simulink library "lib_Conduction_HeatX1DVarPropsAndGenBCs"  (R2015a)
settings: Solver=ode45  StartTime=0.0  StopTime=10.0  RelTol=1e-3
undefined symbols (not defined in the file): dt, T0, x
settings Model: Creator=jlkratz  LastModifiedBy=jlkratz

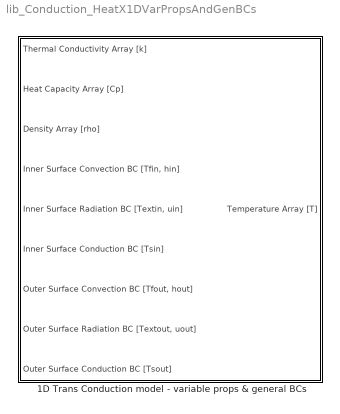
== system lib_Conduction_HeatX1DVarPropsAndGenBCs ==
  1D Trans Conduction model - variable props & general BCs : Subsystem  mask(TSAT: 1-D Trans Conduction Model - Variable Props + Generic BCs Block){x_M=x, T0_M=T0, dt_M=dt, a_M=on, convin_M=on, radin_M=on, condin_M=on, convout_M=on, radout_M=on, condout_M=on, BN_M=double(gcb)}
      mask prompts: x_M "x_M - Discretized spatial domain (node locations) (nx1 array)"; T0_M "T0_M - Initial temperature array (nx1 array)"; dt_M "dt_M - Time step"; a_M "a_M - Shape (unchecked - planar, checked - cylindrical)"; convin_M "convin_M - Convection"; radin_M "radin_M - Radiation"; condin_M "condin_M - Conduction"; convout_M "convout_M - Convection"; radout_M "radout_M - Radiation"; condout_M "condout_M- Conduction"; BN_M "BN_M - Block name"
      mask help:
      | This function models the transient conduction of a 1-D structure which can either be of a planar or cylindrical geometry. This block solves the general 1-D heat equation using a finite difference method. It is able to handle variable thermal properties including density, heat capacity, and thermal conductivity. Abrupt transitions in material are also considered. It has the capability to address dynamic convection, conduction, and radiation boundary conditions. In addition, the discretized domain can be non-uniform but with the restriction that the boundary nodes should be half the thickness of their neighboring interior node (see the help menu).
      |
      | This block is able to accept inputs and parameters in a variety of units but it is important that the units be consistent. More details about this function, it's parameters, inputs, and outputs are provided in the help menu of this block.
      mask init:
      | % Setup Inports ----------------------------------------------------------%
      | 
      | % Inport Numbers
      | n = 4; %first BC inport number
      | 
      | % Inner Suface Convection Boundary Condition
      | if convin_M == 1
      |     if strcmp(get_param([BN_M '/Inner Surface Convection BC [Tfin, hin]'],'BlockType'),'Constant')
      |         MSK_ReplaceBlock_TSAT([BN_M '/Inner Surface Convection BC [Tfin, hin]'],'built-in/Inport');
      |     end
      |     set_param([BN_M '/Inner Surface Convection BC [Tfin, hin]'],'Port',num2str(n));
      |     n = n + 1;
      | elseif convin_M == 0
      |     if strcmp(get_param([BN_M '/Inner Surface Convection BC [Tfin, hin]'],'BlockType'),'Inport')
      |         MSK_ReplaceBlock_TSAT([BN_M '/Inner Surface Convection BC [Tfin, hin]'],'built-in/Constant');
      |         set_param([BN_M '/Inner Surface Convection BC [Tfin, hin]'],'Value','[0, 0]');
      |     end
      | end
      | 
      | % Inner Suface Radiation Boundary Condition
      | if radin_M == 1
      |     if strcmp(get_param([BN_M '/Inner Surface Radiation BC [Textin, uin]'],'BlockType'),'Constant')
      |         MSK_ReplaceBlock_TSAT([BN_M '/Inner Surface Radiation BC [Textin, uin]'],'built-in/Inport');
      |     end
      |     set_param([BN_M '/Inner Surface Radiation BC [Textin, uin]'],'Port',num2str(n));
      |     n = n + 1;
      | elseif radin_M == 0
      |     if strcmp(get_param([BN_M '/Inner Surface Radiation BC [Textin, uin]'],'BlockType'),'Inport')
      |         MSK_ReplaceBlock_TSAT([BN_M '/Inner Surface Radiation BC [Textin, uin]'],'built-in/Constant');
      |         set_param([BN_M '/Inner Surface Radiation BC [Textin, uin]'],'Value','[0, 0]');
      |     end
      | end
      | 
      | % Inner Suface Conduction Boundary Condition
      | if condin_M == 1
      |     if strcmp(get_param([BN_M '/Inner Surface Conduction BC [Tsin]'],'BlockType'),'Constant')
      |         MSK_ReplaceBlock_TSAT([BN_M '/Inner Surface Conduction BC [Tsin]'],'built-in/Inport');
      |     end
      |     set_param([BN_M '/Inner Surface Conduction BC [Tsin]'],'Port',num2str(n));
      |     n = n + 1;
      | elseif condin_M == 0
      |     if strcmp(get_param([BN_M '/Inner Surface Conduction BC [Tsin]'],'BlockType'),'Inport')
      |         MSK_ReplaceBlock_TSAT([BN_M '/Inner Surface Conduction BC [Tsin]'],'built-in/Constant');
      |         set_param([BN_M '/Inner Surface Conduction BC [Tsin]'],'Value','0');
      |     end
      | end
      | 
      | % Outer Suface Convection Boundary Condition
      | if convout_M == 1
      |     if strcmp(get_param([BN_M '/Outer Surface Convection BC [Tfout, hout]'],'BlockType'),'Constant')
      |         MSK_ReplaceBlock_TSAT([BN_M '/Outer Surface Convection BC [Tfout, hout]'],'built-in/Inport');
      |     end
      |     set_param([BN_M '/Outer Surface Convection BC [Tfout, hout]'],'Port',num2str(n));
      |     n = n + 1;
      | elseif convout_M == 0
      |     if strcmp(get_param([BN_M '/Outer Surface Convection BC [Tfout, hout]'],'BlockType'),'Inport')
      |         MSK_ReplaceBlock_TSAT([BN_M '/Outer Surface Convection BC [Tfout, hout]'],'built-in/Constant');
      |         set_param([BN_M '/Outer Surface Convection BC [Tfout, hout]'],'Value','[0, 0]');
      |     end
      | end
      | 
      | % Outer Suface Radiation Boundary Condition
      | if radout_M == 1
      |     if strcmp(get_param([BN_M '/Outer Surface Radiation BC [Textout, uout]'],'BlockType'),'Constant')
      |         MSK_ReplaceBlock_TSAT([BN_M '/Outer Surface Radiation BC [Textout, uout]'],'built-in/Inport');
      |     end
      |     set_param([BN_M '/Outer Surface Radiation BC [Textout, uout]'],'Port',num2str(n));
      |     n = n + 1;
      | elseif radout_M == 0
      |     if strcmp(get_param([BN_M '/Outer Surface Radiation BC [Textout, uout]'],'BlockType'),'Inport')
      |         MSK_ReplaceBlock_TSAT([BN_M '/Outer Surface Radiation BC [Textout, uout]'],'built-in/Constant');
      |         set_param([BN_M '/Outer Surface Radiation BC [Textout, uout]'],'Value','[0, 0]');
      |     end
      | end
      | 
      | % Outer Suface Conduction Boundary Condition
      | if condout_M == 1
      |     if strcmp(get_param([BN_M '/Outer Surface Conduction BC [Tsout]'],'BlockType'),'Constant')
      |         MSK_ReplaceBlock_TSAT([BN_M '/Outer Surface Conduction BC [Tsout]'],'built-in/Inport');
      |     end
      |     set_param([BN_M '/Outer Surface Conduction BC [Tsout]'],'Port',num2str(n));
      |     n = n + 1;
      | elseif condout_M == 0
      |     if strcmp(get_param([BN_M '/Outer Surface Conduction BC [Tsout]'],'BlockType'),'Inport')
      |         MSK_ReplaceBlock_TSAT([BN_M '/Outer Surface Conduction BC [Tsout]'],'built-in/Constant');
      |         set_param([BN_M '/Outer Surface Conduction BC [Tsout]'],'Value','0');
      |     end
      | end
      mask Help: web(which('Conduction_TSAT_1DTCondVarPropGenBC.html'),'-helpbrowser')
      mask DialogControl Container3 Prompt: General Parameters
      mask DialogControl Container4 Prompt: Active Inner Boundary Conditions
      mask DialogControl Container7 Prompt: Active Outer Boundary Conditions

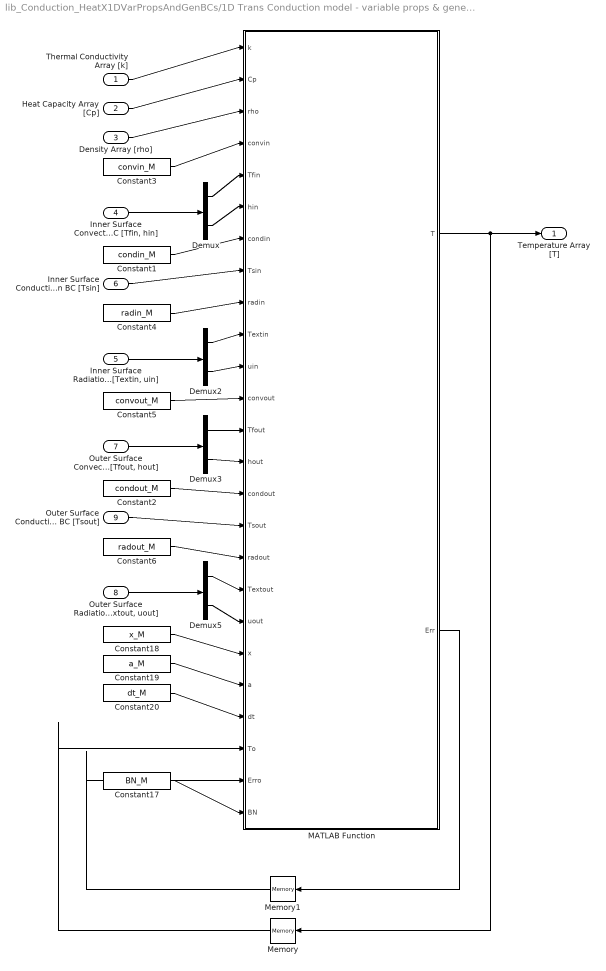
== system lib_Conduction_HeatX1DVarPropsAndGenBCs/1D Trans Conduction model - variable props & general BCs ==
  Thermal Conductivity Array [k] : Inport
  Heat Capacity Array [Cp] : Inport  Port=2
  Density Array [rho] : Inport  Port=3
  "Inner Surface Convection BC [Tfin, hin]" : Inport  Port=4
  "Inner Surface Radiation BC [Textin, uin]" : Inport  Port=5
  Inner Surface Conduction BC [Tsin] : Inport  Port=6
  "Outer Surface Convection BC [Tfout, hout]" : Inport  Port=7
  "Outer Surface Radiation BC [Textout, uout]" : Inport  Port=8
  Outer Surface Conduction BC [Tsout] : Inport  Port=9
  Constant1 : Constant  Value=condin_M
  Constant17 : Constant  Value=BN_M
  Constant18 : Constant  Value=x_M
  Constant19 : Constant  Value=a_M
  Constant2 : Constant  Value=condout_M
  Constant20 : Constant  Value=dt_M
  Constant3 : Constant  Value=convin_M
  Constant4 : Constant  Value=radin_M
  Constant5 : Constant  Value=convout_M
  Constant6 : Constant  Value=radout_M
  Demux{,2..3,5} (4 alike) : Demux  Outputs=[1 1]
  MATLAB Function : MATLAB Function  TreatAsAtomicUnit=on
  Memory : Memory  X0=T0_M
  Memory1 : Memory  X0=zeros(1,37)
  Temperature Array [T] : Outport
  wires:
  "Outer Surface Radiation BC [Textout, uout]"/1 -> Demux5/1
  Demux5/2 -> MATLAB Function/19(uout)
  Demux5/1 -> MATLAB Function/18(Textout)
  Outer Surface Conduction BC [Tsout]/1 -> MATLAB Function/16(Tsout)
  Demux3/2 -> MATLAB Function/14(hout)
  Demux3/1 -> MATLAB Function/13(Tfout)
  "Outer Surface Convection BC [Tfout, hout]"/1 -> Demux3/1
  Demux2/2 -> MATLAB Function/11(uin)
  Demux2/1 -> MATLAB Function/10(Textin)
  "Inner Surface Radiation BC [Textin, uin]"/1 -> Demux2/1
  Inner Surface Conduction BC [Tsin]/1 -> MATLAB Function/8(Tsin)
  Demux/2 -> MATLAB Function/6(hin)
  Demux/1 -> MATLAB Function/5(Tfin)
  "Inner Surface Convection BC [Tfin, hin]"/1 -> Demux/1
  Constant6/1 -> MATLAB Function/17(radout)
  Constant5/1 -> MATLAB Function/12(convout)
  Constant4/1 -> MATLAB Function/9(radin)
  Constant3/1 -> MATLAB Function/4(convin)
  Constant2/1 -> MATLAB Function/15(condout)
  Constant1/1 -> MATLAB Function/7(condin)
  MATLAB Function/2(Err) -> Memory1/1
  Memory/1 -> MATLAB Function/23(To)
  MATLAB Function/1(T) -> Temperature Array [T]/1, Memory/1
  Constant20/1 -> MATLAB Function/22(dt)
  Constant19/1 -> MATLAB Function/21(a)
  Constant18/1 -> MATLAB Function/20(x)
  Density Array [rho]/1 -> MATLAB Function/3(rho)
  Heat Capacity Array [Cp]/1 -> MATLAB Function/2(Cp)
  Thermal Conductivity Array [k]/1 -> MATLAB Function/1(k)
  Memory1/1 -> MATLAB Function/24(Erro)
  Constant17/1 -> MATLAB Function/25(BN)

== matlab function lib_Conduction_HeatX1DVarPropsAndGenBCs/1D Trans Conduction model - variable props & general BCs/MATLAB Function ==
  data: k input; T output; Cp input; rho input; convin input; Tfin input; hin input; condin input; Tsin input; radin input; Textin input; uin input; convout input; Tfout input; hout input; condout input; Tsout input; radout input; Textout input; uout input; x input; a input; dt input; To input; Erro input; Err output; BN input
function [T,Err] = HeatX1D(k,Cp,rho,convin,Tfin,hin,condin,Tsin,...
    radin,Textin,uin,convout,Tfout,hout,condout,Tsout,radout,Textout,uout,...
    x,a,dt,To,Erro,BN)
%#codegen

% Written by: Jonathan Kratz, NASA GRC
% Date: August 1, 2016
%
% Description: This MATLAB function block solves a 1-D heat transfer
% problem with the potential for various boundary conditions including
% convection, conduction, and radiation. The function is capable of
% accepting time-varying thermal properties including the conductivity,
% specific heat, and density of the solid structure. Heat transfer
% coefficients can also be time-varying. The function is equiped to handle
% planor and cylindrical geometries. A generic non-uniform spatial
% discretization may be used but a constant time-step is encouraged for
% accuracy in time. The block applies a 1-D Finite Difference Method (FDM)
% to solve the equation:
%                  _                     _
%   dT     1      |  /dk   ak\ dT     d2T |
%   -- = ------ * | | -- + -- |-- + k --- |
%   dt   rho*Cp   |_ \dx    x/ dx     dx2_|
%
% This is done through the Crank-Nicolson Method in conjunction with 
% Thomas's Algorithm. The boundary conditions use linear heat transfer 
% coefficients and it is suggested that these coefficients be evaluated 
% using thermal properties of the previous time-step (i.e. temperature of 
% the structure and thermodynamic properties of the surrounding gases).
% Depending on the problem they may be assumed constant.
%
% Inputs:
% Thermal Properties:
%   k - thermal conductivity of the structure [1 x number of nodes]
%   Cp - heat capacity of the structure [1 x number of nodes]
%   rho - density of the structure [1 x number of nodes]
% Boundary Conditions:
%   Tfin - temperature of fluid on the inside surface
%   hin - convective heat transfer coefficient on the inside surface
%   Tsin - temperature of a contacting structure on the inside surface
%   Textin - temperature of a distant external radiating source/sink 
%       exposed to the inner surface
%   uin - linear radiative heat transfer coefficient between the inner
%       surface and external radiating source/sink it is exposed to
%   Tfout - temperature of fluid on the outer surface
%   hout - convective heat transfer coefficient on the outer surface
%   Tsout - temperature of a contacting structure on the outer surface
%   Textout - temperature of a distant external radiating source/sink 
%       exposed to the outer surface
%   uin - linear radiative heat transfer coefficient between the outer
%       surface and external radiating source/sink it is exposed to
% Geometry/Discretization:
%   x - discretized spatial coordinates
%   a - shape variable (0 - planar, 1 - cylindrical)
% Solver:
%   dt - time-step of the solver
%   To - initial condition for the solver/initial temperature of the
%       structure [1 x number of nodes]
% Error/Warning Detection
%   Erro - array with error states. Tracks errors/warnings that have been
%       detected.
%   BN - block name. Used in warning messages.
%  
% Discretization guidelines: The first and last nodes should be on the 
% surface. It is important that that the first node should be half the size 
% as the second node and the last node should be half the size of the 
% second to last node. This is due to the assumptions made in the 
% formulization of the boundary condition equations. Also, for planar 
% geometries the first value of the discretization array x (which 
% corresponds to the first node) can be any real numeric value (it does not
% have to be zero, equations use node size so relative position is what 
% matters). In the case of a cylindrical geometry the first value in the x 
% array should be the inner radius of the structure. It should go without 
% saying that the spatial discretization array x is required to be 
% montonically increasing.

% number of elements
n = length(x); %number of nodes

% initialize error/warning array
Err = Erro;
ErrNum = 1; %Error index

% check sizes ------------------------------------------------------------%
if length(x) < 4 && Erro(ErrNum) == 0
    Err(ErrNum) = 1;
    fprintf('warning in %s: x must be an array of length > 3\n',char(BN));
end
ErrNum = ErrNum + 1;
if length(k) ~= length(x) && Erro(ErrNum) == 0
    Err(ErrNum) = 1;
    fprintf('warning in %s: length of k must equal length of x\n',char(BN));
end
ErrNum = ErrNum + 1;
if length(Cp) ~= length(x) && Erro(ErrNum) == 0
    Err(ErrNum) = 1;
    fprintf('warning in %s: length of k must equal length of x\n',char(BN));
end
ErrNum = ErrNum + 1;
if length(rho) ~= length(x) && Erro(ErrNum) == 0
    Err(ErrNum) = 1;
    fprintf('warning in %s: length of k must equal length of x\n',char(BN));
end
ErrNum = ErrNum + 1;
if length(x) ~= length(x) && Erro(ErrNum) == 0
    Err(ErrNum) = 1;
    fprintf('warning in %s: length of k must equal length of x\n',char(BN));
end
ErrNum = ErrNum + 1;
if length(Tfin) ~= 1 && Erro(ErrNum) == 0
    Err(ErrNum) = 1;
    fprintf('warning in %s: Tfin must be a scalar\n',char(BN));
end
ErrNum = ErrNum + 1;
if length(hin) ~= 1 && Erro(ErrNum) == 0
    Err(ErrNum) = 1;
    fprintf('warning in %s: hin must be a scalar\n',char(BN));
end
ErrNum = ErrNum + 1;
if length(Tsin) ~= 1 && Erro(ErrNum) == 0
    Err(ErrNum) = 1;
    fprintf('warning in %s: Tsin must be a scalar\n',char(BN));
end
ErrNum = ErrNum + 1;
if length(Textin) ~= 1 && Erro(ErrNum) == 0
    Err(ErrNum) = 1;
    fprintf('warning in %s: Textin must be a scalar\n',char(BN));
end
ErrNum = ErrNum + 1;
if length(uin) ~= 1 && Erro(ErrNum) == 0
    Err(ErrNum) = 1;
    fprintf('warning in %s: uin must be a scalar\n',char(BN));
end
ErrNum = ErrNum + 1;
if length(Tfout) ~= 1 && Erro(ErrNum) == 0
    Err(ErrNum) = 1;
    fprintf('warning in %s: Tfout must be a scalar\n',char(BN));
end
ErrNum = ErrNum + 1;
if length(hout) ~= 1 && Erro(ErrNum) == 0
    Err(ErrNum) = 1;
    fprintf('warning in %s: hout must be a scalar\n',char(BN));
end
ErrNum = ErrNum + 1;
if length(Tsout) ~= 1 && Erro(ErrNum) == 0
    Err(ErrNum) = 1;
    fprintf('warning in %s: Tsout must be a scalar\n',char(BN));
end
ErrNum = ErrNum + 1;
if length(Textout) ~= 1 && Erro(ErrNum) == 0
    Err(ErrNum) = 1;
    fprintf('warning in %s: Textout must be a scalar\n',char(BN));
end
ErrNum = ErrNum + 1;
if length(uout) ~= 1 && Erro(ErrNum) == 0
    Err(ErrNum) = 1;
    fprintf('warning in %s: uin must be a scalar\n',char(BN));
end
ErrNum = ErrNum + 1;
if ((length(a) ~= 1) || (a ~= 0 && a ~= 1)) && Erro(ErrNum) == 0
    Err(ErrNum) = 1;
    fprintf('warning in %s: a must be a scalar equal to 0 or 1\n',char(BN));
end
ErrNum = ErrNum + 1;
if (length(dt) ~= 1 || dt <= 0) && Erro(ErrNum) == 0
    Err(ErrNum) = 1;
    fprintf('warning in %s: dt must be a positive scalar\n',char(BN));
end
ErrNum = ErrNum + 1;

% check for physical impossibilities
if min(k) <= 0 && Erro(ErrNum) == 0
    Err(ErrNum) = 1;
    fprintf('warning in %s: elements of k cannot be zero or negative\n',char(BN));
end
ErrNum = ErrNum + 1;
if min(Cp) <= 0 && Erro(ErrNum) == 0
    Err(ErrNum) = 1;
    fprintf('warning in %s: elements of Cp cannot be zero or negative\n',char(BN));
end
ErrNum = ErrNum + 1;
if min(rho) <= 0 && Erro(ErrNum) == 0
    Err(ErrNum) = 1;
    fprintf('warning in %s: elements of rho cannot be zero or negative\n',char(BN));
end
ErrNum = ErrNum + 1;
if min(To) < 0 && Erro(ErrNum) == 0
    Err(ErrNum) = 1;
    fprintf('warning in %s: elements of T0 are negative. On an absolute scale this is not possible.\n',char(BN));
end
ErrNum = ErrNum + 1;
if Tfin < 0 && Erro(ErrNum) == 0
    Err(ErrNum) = 1;
    fprintf('warning in %s: Tfin is negative. On an absolute scale this is not possible.\n',char(BN));
end
ErrNum = ErrNum + 1;
if Tfout < 0 && Erro(ErrNum) == 0
    Err(ErrNum) = 1;
    fprintf('warning in %s: Tfout is negative. On an absolute scale this is not possible.\n',char(BN));
end
ErrNum = ErrNum + 1;
if Tsin < 0 && Erro(ErrNum) == 0
    Err(ErrNum) = 1;
    fprintf('warning in %s: Tsin is negative. On an absolute scale this is not possible.\n',char(BN));
end
ErrNum = ErrNum + 1;
if Tsout < 0 && Erro(ErrNum) == 0
    Err(ErrNum) = 1;
    fprintf('warning in %s: Tsout is negative. On an absolute scale this is not possible.\n',char(BN));
end
ErrNum = ErrNum + 1;
if Textin < 0 && Erro(ErrNum) == 0
    Err(ErrNum) = 1;
    fprintf('warning in %s: Textin is negative. On an absolute scale this is not possible.\n',char(BN));
end
ErrNum = ErrNum + 1;
if Textout < 0 && Erro(ErrNum) == 0
    Err(ErrNum) = 1;
    fprintf('warning in %s: Textout is negative. On an absolute scale this is not possible.\n',char(BN));
end
ErrNum = ErrNum + 1;
if hin < 0 && Erro(ErrNum) == 0
    Err(ErrNum) = 1;
    fprintf('warning in %s: hin must be positive.\n',char(BN));
end
ErrNum = ErrNum + 1;
if hout < 0 && Erro(ErrNum) == 0
    Err(ErrNum) = 1;
    fprintf('warning in %s: hout must be positive.\n',char(BN));
end
ErrNum = ErrNum + 1;
if uin < 0 && Erro(ErrNum) == 0
    Err(ErrNum) = 1;
    fprintf('warning in %s: uin must be positive.\n',char(BN));
end
ErrNum = ErrNum + 1;
if uout < 0 && Erro(ErrNum) == 0
    Err(ErrNum) = 1;
    fprintf('warning in %s: uout must be positive.\n',char(BN));
end
ErrNum = ErrNum + 1;

% check for defiance of block constraints
diffx = diff(x);
if min(diffx) <= 0 && Erro(ErrNum) == 0
    Err(ErrNum) = 1;
    fprintf('warning in %s: x must be monotonically increasing\n',char(BN));
end
ErrNum = ErrNum + 1;
if (x(2)-x(1))-(x(3)-x(2)) >= 10^-5 && Erro(ErrNum) == 0
    x(1)
    x(2)
    x(3)
    Err(ErrNum) = 1;
    fprintf('warning in %s: the first node may not be half the thickness of the\nneighboring interior node as is required for planar geometries in the\nequation formulation of this block. To assure the first node is\nof the appropriate size assure (x(2)-x(1))-(x(3)-x(2)) = 0.\n',char(BN));
end
ErrNum = ErrNum + 1;
if (x(n)-x(n-1))-(x(n-1)-x(n-2)) >= 10^-5 && Erro(ErrNum) == 0
    Err(ErrNum) = 1;
    fprintf('warning in %s: the last node may not be half the thickness of the\nneighboring interior node as is required for planar geometries in the\nequation formulation of this block. To assure the last node is\nof the appropriate size assure (x(n)-x(n-1))-(x(n-1)-x(n-2)) = 0\nwhere n is the total number of nodes.\n',char(BN));
end
ErrNum = ErrNum + 1;
if a == 1 && x(1) < 10^-6 %protect against dividing by zero
    if Erro(ErrNum) == 0
        fprintf('warning in %s: x(1) is close to zero, value changed to 10^-6 to prevent dividing by zero\n',char(BN));
    end
    Err(ErrNum) = 1;
    x(1) = 10^-6;
end
ErrNum = ErrNum + 1;

% verify at least one BC type is active for each surface
if condin == 0 && convin == 0 && radin == 0 && Erro(ErrNum) == 0
    fprintf('warning in %s: at least one boundary condition type (convection, radiation, conduction) must be active for the inner surface\n',char(BN));
    Err(ErrNum) = 1;
end
ErrNum = ErrNum + 1;
% verify at least one BC type is active for each surface
if condout == 0 && convout == 0 && radout == 0 && Erro(ErrNum) == 0
    fprintf('warning in %s: at least one boundary condition type (convection, radiation, conduction) must be active for the outer surface\n',char(BN));
    Err(ErrNum) = 1;
end

% make external convection at boundaries zero if there is no convection BC
if convin == 0
    hin = 0;
end
if convout == 0
    hout = 0;
end

% make external radiation at boundaries zero if there is no radiation BC
if radin == 0
    uin = 0;
end
if radout == 0
    uout = 0;
end

% form system of equations in tridiagonal arrays -------------------------%
%  _                                 _  _   _     _   _ 
% | D1   A1   0    .    .    .    0   || T1  |   | C1  |
% | B1   D2   A2   0              .   || T2  |   | C2  |
% | 0    B2   D3   A3   .         .   || T3  |   | C3  |
% | .    0    .    .    .    .    .   || .   | = | .   |
% | .         .    .    .    .    0   || .   |   | .   | 
% | .              .    Bn-2 Dn-1 An-1|| Tn-1|   | Cn-1|
% |_0    .    .    .    0    Bn-1 Dn _||_Tn _|   |_Cn _|
%
% Initialize system arrays B, D, A, and C
B = zeros(1,n); %initialize B array
D = zeros(1,n); %initialize D array
A = zeros(1,n); %initialize A array
C = zeros(1,n); %initialize C array
% node thickness
dx = zeros(1,n); %initialize dx array
for i = 1:n
    if i == 1
        dx(i) = (x(2)-x(1));
    elseif i == n
        dx(i) = (x(n)-x(n-1));
    else
        del1 = x(i) - x(i-1);
        dx(i) = 2*del1 - dx(i-1);
    end
end
% --- inner node (half size of interior node with point on surface)
Fo1 = 0; %Fourier number
Bi1 = 0; %Boit number
BiRad1 = 0; %analogous Boit number for radiation
Fos1 = 0; %Fourier number for conduction BC
dx1 = x(2) - x(1); %node size
% planar
if a == 0
    Fo1 = dt*k(1)/(rho(1)*Cp(1)*dx1^2); %Fourier number
    Bi1 = hin*dx1/k(1); %Boit number
    BiRad1 = uin*dx1/k(1); %analogous Boit number for radiation
    if condin == 0
        Fos1 = 0;
    else
        Fos1 = Fo1/(10^-4); %Fourier number for conduction BC
    end
end
% cylindrical
if a == 1
    Fo1 = dt*k(1)/(rho(1)*Cp(1)*((x(2)-dx1/2)^2-x(1)^2)*log(x(2)/x(1))); %Fourier number
    Bi1 = hin*x(1)*log(x(2)/x(1))/k(1); %Boit number
    BiRad1 = uin*x(1)*log(x(2)/x(1))/k(1); %analogous Boit number for radiation
    if condin == 0
        Fos1 = 0;
    else
        if (x(1)-dx1) <= 0
            dx1 = 0;
        end
        Fos1 = dt*k(1)/(rho(1)*Cp(1)*((x(2)-dx1/2)^2-x(1)^2)*log((x(1)/(x(1)-dx1))))/(10^-4); %Fourier number for conduction BC
    end
end
% form system arrays
B(1) = 0;
D(1) = 1 + Fo1 + Fo1*Bi1 + Fo1*BiRad1 + Fos1; %system array D
A(1) = -Fo1; %system array A
C(1) = (1 - Fo1 - Fo1*Bi1 - Fo1*BiRad1 - Fos1)*To(1) + Fo1*To(2) + 2*Fo1*Bi1*Tfin + 2*Fo1*BiRad1*Textin + 2*Fos1*Tsin; %system array C
% --- interior nodes
for i = 2:(n-1)
    % distance between nodes
    del1 = x(i) - x(i-1);
    del2 = x(i+1) - x(i);
    % simplification coefficients (for spatial discretization)
    C1 = 1 + (del1^3/del2^2 - del1)/(del2 + del1);
    C2 = 1 + (del1/del2)^3;
    C3 = (del1/del2)^3 - ((del1^3/del2^2) - del1)/(del2+del1);
    % calculated Fourier numbers
    Fo = 2*k(i)*dt/(rho(i)*Cp(i)*(del1^2 + del1^3/del2)); %Fourier number
    Fok = (dt/(rho(i)*Cp(i)*(del1+del2)))*((k(i+1)-k(i-1))/(del1+del2) + a*k(i)/x(i)); %Fourier number for conductivity variation and shape
    % adjust equations for change in materials
    %   when there is a change in materials the transition in materials
    %   properties, most notabely thermal conductivity, is abrupt. This
    %   discontinuty can cause accuracy and stability issues with the 
    %   derivative term dk/dt = (k(i+1)-k(i-1))/(del1+del2). Therefore a
    %   more robust approach is utilized when a material transition is
    %   detected. This method is document in "Integrated Turbine Tip
    %   Clearance and Gas Turbine Engine Simulation" by J. Chapman, J.
    %   Kratz, T.-H. Guo, and J. Litt. The method uses a transition Fourier
    %   number to address the discontinuity. The method from this reference
    %   has been generalized for non-uniform discretizations and geometries
    %   that could be either planar or cylindrical. When there is not a
    %   transition in materials the dk/dt term should be better
    %   approximated with the central difference scheme that is used and
    %   the standard formulation will be utilized. Material transition is
    %   detected by a sigificant (10%) increase or decrease in thermal 
    %   conductivity.
    if (k(i+1)/k(i)) > 1.1 || (k(i+1)/k(i)) < 0.9 %detect change in material
        Fo = k(i)*dt/(rho(i)*Cp(i)*dx(i)^2);
        Fok = (dt/(rho(i)*Cp(i)*(del1+del2)))*(a*k(i)/x(i));
        Fob = (k(i)*(dx(i)/2)+k(i+1)*(del2-dx(i)/2))*dt/(rho(i)*Cp(i)*del2*del1*del2);
        K1 = Fo;
        K2 = 2*0.5*(Fo+Fob); 
        K3 = Fob;
    elseif (k(i)/k(i-1)) > 1.1 || (k(i)/k(i-1)) < 0.9 %detect change in material
        Fo = k(i)*dt/(rho(i)*Cp(i)*dx(i)^2);
        Fok = (dt/(rho(i)*Cp(i)*(del1+del2)))*(a*k(i)/x(i));
        Foa = (k(i)*(dx(i)/2)+k(i-1)*(del1-dx(i)/2))*dt/(rho(i)*Cp(i)*del1*del1*del2);
        K1 = Foa;
        K2 = 2*0.5*(Fo+Foa); 
        K3 = Fo;
    else % no change in material detected - go with standard solution
        K1 = C1*Fo;
        K2 = C2*Fo;
        K3 = C3*Fo;
    end
    % form system arrays (B, D, A, and C)
    B(i) = 0.5*Fok - 0.5*K1;
    D(i) = 1 + 0.5*K2;
    A(i) = -0.5*Fok - 0.5*K3;
    C(i) = (-0.5*Fok+0.5*K1)*To(i-1) + (1-0.5*K2)*To(i) + (0.5*Fok+0.5*K3)*To(i+1);
end
% --- outer node (half size of interior node with point on surface)
Fon = 0; %Fourier number
Bin = 0; %Boit number
BiRadn = 0; %analogous Boit number for radiation
Fosn = 0; %Fourier number for conduction BC
dxn = x(n) - x(n-1); %node size
% planar
if a == 0
    Fon = dt*k(n)/(rho(n)*Cp(n)*dxn^2); %Fourier number
    Bin = hout*dxn/k(n); %Boit number
    BiRadn = uout*dxn/k(n); %analogous Boit number for radiation
    if condout == 0
        Fosn = 0;
    else
        Fosn = Fon/(10^-4); %Fourier number for conduction BC
    end
end
% cylindrical
if a == 1
    Fon = dt*k(n)/(rho(n)*Cp(n)*(x(n)^2-(x(n-1)+dxn/2)^2)*log(x(n)/x(n-1))); %Fourier number
    Bin = hout*x(n)*log(x(n)/x(n-1))/k(n); %Boit number
    BiRadn = uout*x(n)*log(x(n)/x(n-1))/k(n); %analogous Boit number for radiation
    if condout == 0
        Fosn = 0;
    else
        Fosn = dt*k(n)/(rho(n)*Cp(n)*(x(n)^2-(x(n-1)+dxn/2)^2)*log((x(n)+dxn)/x(n)))/(10^-4); %Fourier number for conduction BC
    end
end
% form system arrays
D(n) = 1 + Fon + Fon*Bin + Fon*BiRadn + Fosn; %system array D
B(n) = -Fon; %system array B
A(n) = 0; %system array A
C(n) = (1 - Fon - Fon*Bin - Fon*BiRadn - Fosn)*To(n) + Fon*To(n-1) + 2*Fon*Bin*Tfout + 2*Fon*BiRadn*Textout + 2*Fosn*Tsout; %system array C

% solve for new temperatures using Thomas's Algorithm --------------------%
Dnew = zeros(1,n);
Cnew = zeros(1,n);
Dnew(1) = D(1);
Cnew(1) = C(1);
% build the rest of the new D-vector and C-vector using Guassian
% elimination
for i = 2:n
    Dnew(i) = D(i) - A(i-1)*B(i)/Dnew(i-1);
    Cnew(i) = C(i) - B(i)*Cnew(i-1)/Dnew(i-1);
end
% initialize the solution vector (i.e. the new temperature vector T)
T = zeros(1,n);
T(n) = Cnew(n)/Dnew(n);
for i = (n-1):-1:1
    T(i) = (Cnew(i) - A(i)*T(i+1))/Dnew(i);
end
